simulink model "RO_Process_V1"  (R2021b)
settings: Solver=VariableStepAuto  StartTime=0.0  StopTime=10000  MaxStep=1  RelTol=1e-3
values from neighbouring files (symbols this model uses):
  A0 = 5.501e-7    (= 5.501e-07)    [main_V1.m]
  aT = 3    [main_V1.m]
  B0 = 1.82e-5    (= 1.82e-05)    [main_V1.m]
  bT = 3.08    [main_V1.m]
  Cf = 20    [main_V1.m]
  d0 = 84e-6    (= 8.4e-05)    [main_V1.m]
  di = 42e-6    (= 4.2e-05)    [main_V1.m]
  eta = .01    (= 0.01)    [main_V1.m]
  Ff = 1    [main_V1.m]
  l = 2    [main_V1.m]
  Lb = 32*eta_b*lb^2/(di^2*Pmax)    (= 16.4914450629)    [main_V1.m]
  Lm = 32*eta_m*lm^2/(dm^4*Pmax)    (= 584305734.937)    [main_V1.m]
  ls = 2    [main_V1.m]
  Pf = 8000    [main_V1.m]
  phi_b = 128*eta_b*lb/(pi*ro_b*di^2)    (= 923.892640171)    [main_V1.m]
  R = 8.314    [main_V1.m]
  ro_p = 50    [main_V1.m]
  T0 = 291    [main_V1.m]
  Tf = 303    [main_V1.m]
settings Model: Creator=Arash  LastModifiedBy=Arash
settings SolverCC: AlgebraicLoopSolver=TrustRegion
settings DataIOCC: ReturnWorkspaceOutputs=off
settings DebuggingCC: SFMachineParentedDataDiag=warning  ArithmeticOperatorsInVariantConditions=warning
settings SFSimCC: CustomCodeUndefinedFunction=UseInterfaceOnly

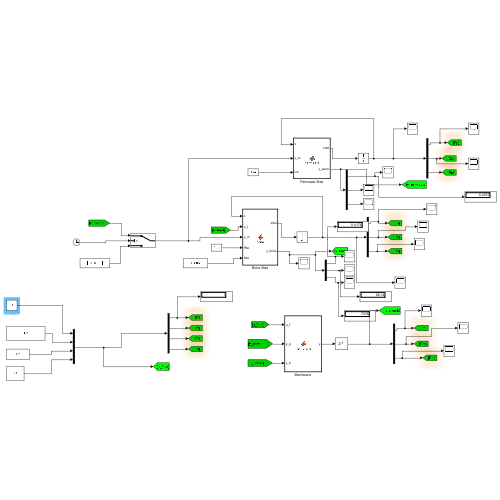
[thumbnail: Simulink's stored preview of the top-level diagram]
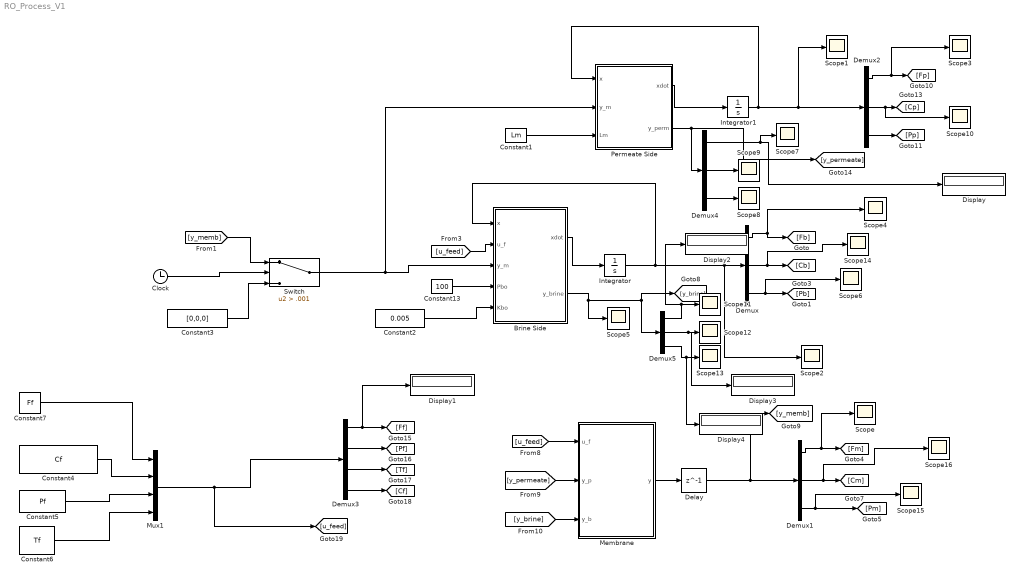
== system RO_Process_V1 ==
  Brine Side : MATLAB Function  TreatAsAtomicUnit=on
  Clock : Clock
  Constant1 : Constant  Value=Lm
  Constant13 : Constant  Value=100
  Constant2 : Constant  Value=0.005
  Constant3 : Constant  Value=[0,0,0]
  Constant4 : Constant  Value=Cf
  Constant5 : Constant  Value=Pf
  Constant6 : Constant  Value=Tf
  Constant7 : Constant  Value=Ff
  Delay : Delay  DelayLength=1
  Demux{,1..2,4..5} (5 alike) : Demux  Outputs=3
  Demux3 : Demux
  Display{,1..4} (5 alike) : Display
  Integrator : Integrator  InitialCondition=[1e2;10;2000]
  Integrator1 : Integrator  InitialCondition=[1e1;0;100]
  "Membrane " : MATLAB Function  TreatAsAtomicUnit=on
  Mux1 : Mux
  Permeate Side : MATLAB Function  TreatAsAtomicUnit=on
  Scope{,1..16} (17 alike) : Scope
  Switch : Switch  Criteria=u2 > Threshold  Threshold=.001
  wires:
  Demux/1 -> Scope4/1, [Fb]
  Demux/2 -> [Cb], Scope14/1
  Brine Side/1(xdot) -> Integrator/1
  Integrator/1 -> Brine Side/1(x), Scope2/1, Demux/1
  Permeate Side/1(xdot) -> Integrator1/1
  [u_feed] -> Brine Side/2(u_f)
  Demux1/1 -> Scope/1, [Fm]
  Demux2/1 -> Scope3/1, [Fp]
  Integrator1/1 -> Scope1/1, Demux2/1, Permeate Side/1(x)
  Switch/1 -> Permeate Side/2(y_m), Brine Side/3(y_m)
  Constant1/1 -> Permeate Side/3(Lm)
  Constant13/1 -> Brine Side/4(Pbo)
  [u_feed] -> "Membrane "/1(u_f)
  [y_permeate] -> "Membrane "/2(y_p)
  [y_brine] -> "Membrane "/3(y_b)
  Demux3/3 -> [Tf]
  Demux3/2 -> [Pf]
  Demux3/4 -> [Cf]
  Demux3/1 -> Display1/1, [Ff]
  "Membrane "/1(y) -> Delay/1
  Brine Side/2(y_brine) -> Demux5/1, [y_brine], Scope5/1
  Constant3/1 -> Switch/3
  [y_memb] -> Switch/1
  Clock/1 -> Switch/2
  Demux/3 -> [Pb], Scope6/1
  Delay/1 -> [y_memb], Demux1/1
  Permeate Side/2(y_perm) -> Demux4/1, [y_permeate]
  Demux4/3 -> Scope8/1
  Demux4/2 -> Scope9/1
  Demux4/1 -> Display/1, Scope7/1
  Demux5/1 -> Scope11/1, Display2/1
  Demux5/2 -> Display3/1, Scope12/1
  Demux5/3 -> Display4/1, Scope13/1
  Constant2/1 -> Brine Side/5(Kbo)
  Demux2/2 -> Scope10/1, [Cp]
  Demux2/3 -> [Pp]
  Demux1/3 -> [Pm], Scope15/1
  Demux1/2 -> Scope16/1, [Cm]
  Mux1/1 -> [u_feed], Demux3/1
  Constant4/1 -> Mux1/2
  Constant5/1 -> Mux1/3
  Constant6/1 -> Mux1/4
  Constant7/1 -> Mux1/1

== matlab function RO_Process_V1/Brine Side ==
  data: x input; u_f input; xdot output; y_m input; Pbo input; Lb parameter; phi_b parameter; y_brine output; Kbo input
function [xdot,y_brine] = brine(x,u_f,y_m,Pbo,Lb, phi_b, Kbo)
% Feed water stream
Ff=u_f(1);
Cf=u_f(2);
Pf=u_f(3);
Tf=u_f(4);

% Membrane stream
Fm=y_m(1);
Cm=y_m(2);
Pm=y_m(3);
% states of brine
mb=x(1);
Cb=x(2);
Pb=x(3);
Fb=Kbo*sqrt(Pb-Pbo);
mb_dot=Ff-Fb-Fm;
if (Fb+Fm)>Ff
   Fb=Ff-Fm; 
end
Cb_dot=1/mb*(Ff*(Cf-Cb)-Fm*(.01*Cm-Cb));
Pb_dot=1/Lb*(Pf-Pb-phi_b*Ff);
xdot=[mb_dot;Cb_dot;Pb_dot];

y_brine=[Fb;x(2);Pb];

== matlab function RO_Process_V1/Permeate Side ==
  data: x input; y_m input; Lm input; xdot output; phi_m parameter; y_perm output
function [xdot,y_perm] = permeate(x,y_m,Lm, phi_m)

% Membrane stream
Fm=y_m(1);
Cm=y_m(2);
Pm=y_m(3);
% states of brine
mp=x(1);
Cp=x(2);
Pp=x(3);

mp_dot=0;

Cp_dot=Fm/mp*(Cm-Cp);
Pp_dot=1/Lm*(-Pp+phi_m*Fm);
xdot=[mp_dot;Cp_dot;Pp_dot];
y_perm=[Fm;x(2);x(3)];

== matlab function RO_Process_V1/Membrane  ==
  data: u_f input; y_p input; y output; y_b input; R parameter; ls parameter; l parameter; ro_p parameter; A0 parameter; B0 parameter; T0 parameter; aT parameter; bT parameter; eta parameter; d0 parameter; di parameter
function y = membrane(u_f,y_p,y_b,R, ls, l, ro_p, A0, B0, T0, aT, bT, eta, d0, di)
%Feed stream
Fb=y_b(1);
Cb=y_b(2);
Pb=y_b(3);
%Brine stream
Fp=y_p(1);
Cp=y_p(2);
Pp=y_p(3);
% Membrane stream
Ff=u_f(1);
Cf=u_f(2);
Pf=u_f(3);
Tf=u_f(4);
A=A0*exp(aT*(Tf-T0)/Tf);
B=B0*exp(bT*(Tf-T0)/Tf);
pi_b=75.84*Cb;
pi_p=75.84*Cp;
pi_f=75.84*Cf;
delta_pi=(pi_f+pi_b)/2-pi_p;
delta_p=(Pf+Pb)/2-Pp;
% output of membrane
% H=sqrt(128*eta*d0*A/di^4);
% Fm=A*ro_p*(delta_p-delta_pi)*tanh(H*l)/(H+H^2*ls*tanh(H*l))+B*(Cf-Cp);
Cm=Cb;

Fm=A*ro_p*(delta_p-delta_pi)+B*(Cf-Cp);

y=[Fm;Cm;Pp];
